simulink model "simple_router"  (R2015a)
settings: Solver=ode45  StartTime=0.0  StopTime=3000  FixedStep=1  RelTol=1e-3
undefined symbols (not defined in the file or in its folder): des, SELECT, T
libraries: simulink x16
(part 1 of 6)
settings Model: CovSFcnEnable=off  Creator=Nejib  LastModifiedBy=Nejib
settings DebuggingCC: SolverPrmCheckMsg=warning
settings SimEventsCC: propMaxDesBlkSimulEvents=100000  propMaxDesMdlSimulEvents=10000000

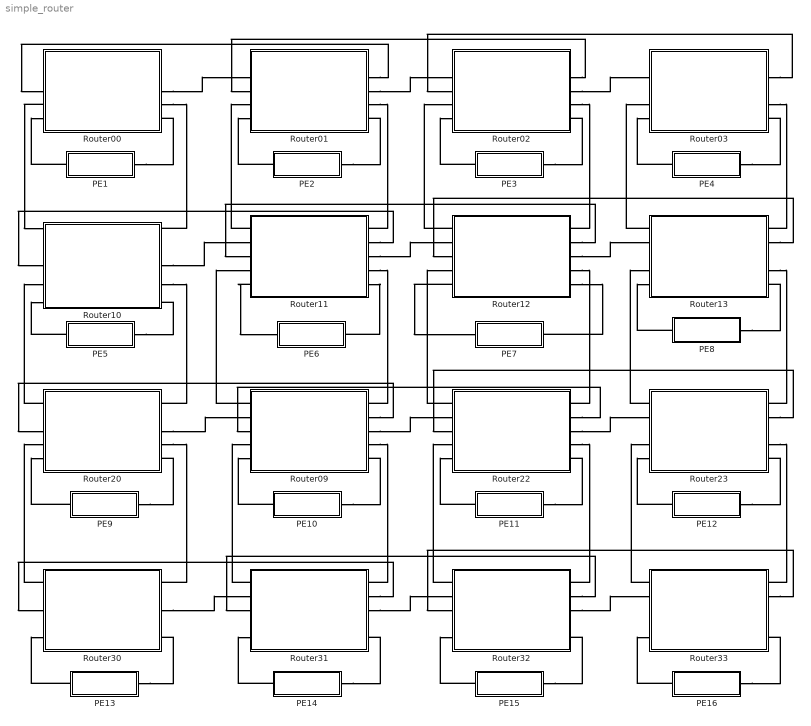
== system simple_router ==
  PE1 : Subsystem  mask{ME=1, D=5, SEED=100, tt=Periodic, MINU=10, MAXU=200, REGULAR=T, A=100, B=15, Inst='Inst1', Router='Mean1', Loss='Loss1', N='N1'}
      mask prompts: ME "Adresse"; D "Startup time"; tt "Traffic Type"; MINU "Min"; MAXU "Max"; REGULAR "T"; A "Lambda 1"; B "Lambda 2"; Inst "Instant delay"; Router "Mean delay"; Loss "Instant number of lost flits"; N "Number of departed flits"
      mask init:
      | set_param([gcb '/Inst'],'VariableName',Inst)
      | set_param([gcb '/Router'],'VariableName',Router)
      | set_param([gcb '/Loss'],'VariableName',Loss)
      | set_param([gcb '/N'],'VariableName',N)
      | V=1:16;
      | V=V(V~=ME);
      mask TypeOptions tt: Periodic | Uniform | MMPP
      mask Callback tt:
      | maskStr = get_param(gcb,'tt');
      | msk = Simulink.Mask.get(gcbh);
      | %p = msk.Parameters;
      | %
      | % P = msk.getParameter('MINU');
      | % U = msk.getParameter('MAXU');
      | % M = msk.getParameter('REGULAR');
      | 
      | P = msk.getDialogControl('Periodic');
      | U = msk.getDialogControl('Uniform');
      | M = msk.getDialogControl('MMPP');
      | 
      | % The pop-up menu is the first mask parameter.
      | %   Check the value selected in the pop-up
      | if strcmp(maskStr(1),'P'),
      | 
      |     % Set the visibility of both parameters on when
      |     %   User-defined is selected in the pop-up.
      |     %set_param(gcb,'MaskValues',{'Default','1','1'})
      |     %set_param(gcb,'MaskVisibilities','off'),
      |     SELECT = 1;
      |     P.Visible= 'on';
      |     U.Visible= 'off';
      |     M.Visible= 'off';
      | 
      | elseif strcmp(maskStr(1),'U'),
      |     P.Visible= 'off';
      |     U.Visible= 'on';
      |     M.Visible= 'off';
      | 
      |     SELECT = 2;
      | else
      |     P.Visible= 'off';
      |     U.Visible= 'off';
      |     M.Visible= 'on';
      | 
      |     SELECT = 3;
      | end
      mask DialogControl DescTextVar Prompt: Generates traffic from a given adress using one of three possible traffic patterns: Periodic, Uniform and Markov Modulated Poisson Process.
  PE10 : Subsystem  mask{ME=10, D=5, SEED=1000, tt=Periodic, MINU=10, MAXU=200, REGULAR=T, A=100, B=15, Inst='Inst10', Router='Mean10', Loss='Loss10', N='N10'}
      mask prompts: ME "Adresse"; D "Startup time"; tt "Traffic Type"; MINU "Min"; MAXU "Max"; REGULAR "T"; A "Lambda 1"; B "Lambda 2"; Inst "Instant delay"; Router "Mean delay"; Loss "Instant number of lost flits"; N "Number of departed flits"
      mask init:
      | set_param([gcb '/Inst'],'VariableName',Inst)
      | set_param([gcb '/Router'],'VariableName',Router)
      | set_param([gcb '/Loss'],'VariableName',Loss)
      | set_param([gcb '/N'],'VariableName',N)
      | V=1:16;
      | V=V(V~=ME);
      mask TypeOptions tt: Periodic | Uniform | MMPP
      mask Callback tt:
      | maskStr = get_param(gcb,'tt');
      | msk = Simulink.Mask.get(gcbh);
      | %p = msk.Parameters;
      | %
      | % P = msk.getParameter('MINU');
      | % U = msk.getParameter('MAXU');
      | % M = msk.getParameter('REGULAR');
      | 
      | P = msk.getDialogControl('Periodic');
      | U = msk.getDialogControl('Uniform');
      | M = msk.getDialogControl('MMPP');
      | 
      | % The pop-up menu is the first mask parameter.
      | %   Check the value selected in the pop-up
      | if strcmp(maskStr(1),'P'),
      | 
      |     % Set the visibility of both parameters on when
      |     %   User-defined is selected in the pop-up.
      |     %set_param(gcb,'MaskValues',{'Default','1','1'})
      |     %set_param(gcb,'MaskVisibilities','off'),
      |     SELECT = 1;
      |     P.Visible= 'on';
      |     U.Visible= 'off';
      |     M.Visible= 'off';
      | 
      | elseif strcmp(maskStr(1),'U'),
      |     P.Visible= 'off';
      |     U.Visible= 'on';
      |     M.Visible= 'off';
      | 
      |     SELECT = 2;
      | else
      |     P.Visible= 'off';
      |     U.Visible= 'off';
      |     M.Visible= 'on';
      | 
      |     SELECT = 3;
      | end
      mask DialogControl DescTextVar Prompt: Generates traffic from a given adress using one of three possible traffic patterns: Periodic, Uniform and Markov Modulated Poisson Process.
  PE11 : Subsystem  mask{ME=11, D=5, SEED=1100, tt=Periodic, MINU=10, MAXU=200, REGULAR=T, A=100, B=15, Inst='Inst11', Router='Mean11', Loss='Loss11', N='N11'}
      mask prompts: ME "Adresse"; D "Startup time"; tt "Traffic Type"; MINU "Min"; MAXU "Max"; REGULAR "T"; A "Lambda 1"; B "Lambda 2"; Inst "Instant delay"; Router "Mean delay"; Loss "Instant number of lost flits"; N "Number of departed flits"
      mask init:
      | set_param([gcb '/Inst'],'VariableName',Inst)
      | set_param([gcb '/Router'],'VariableName',Router)
      | set_param([gcb '/Loss'],'VariableName',Loss)
      | set_param([gcb '/N'],'VariableName',N)
      | V=1:16;
      | V=V(V~=ME);
      mask TypeOptions tt: Periodic | Uniform | MMPP
      mask Callback tt:
      | maskStr = get_param(gcb,'tt');
      | msk = Simulink.Mask.get(gcbh);
      | %p = msk.Parameters;
      | %
      | % P = msk.getParameter('MINU');
      | % U = msk.getParameter('MAXU');
      | % M = msk.getParameter('REGULAR');
      | 
      | P = msk.getDialogControl('Periodic');
      | U = msk.getDialogControl('Uniform');
      | M = msk.getDialogControl('MMPP');
      | 
      | % The pop-up menu is the first mask parameter.
      | %   Check the value selected in the pop-up
      | if strcmp(maskStr(1),'P'),
      | 
      |     % Set the visibility of both parameters on when
      |     %   User-defined is selected in the pop-up.
      |     %set_param(gcb,'MaskValues',{'Default','1','1'})
      |     %set_param(gcb,'MaskVisibilities','off'),
      |     SELECT = 1;
      |     P.Visible= 'on';
      |     U.Visible= 'off';
      |     M.Visible= 'off';
      | 
      | elseif strcmp(maskStr(1),'U'),
      |     P.Visible= 'off';
      |     U.Visible= 'on';
      |     M.Visible= 'off';
      | 
      |     SELECT = 2;
      | else
      |     P.Visible= 'off';
      |     U.Visible= 'off';
      |     M.Visible= 'on';
      | 
      |     SELECT = 3;
      | end
      mask DialogControl DescTextVar Prompt: Generates traffic from a given adress using one of three possible traffic patterns: Periodic, Uniform and Markov Modulated Poisson Process.
  PE12 : Subsystem  mask{ME=12, D=5, SEED=1200, tt=Periodic, MINU=10, MAXU=200, REGULAR=T, A=100, B=15, Inst='Inst12', Router='Mean12', Loss='Loss12', N='N12'}
      mask prompts: ME "Adresse"; D "Startup time"; tt "Traffic Type"; MINU "Min"; MAXU "Max"; REGULAR "T"; A "Lambda 1"; B "Lambda 2"; Inst "Instant delay"; Router "Mean delay"; Loss "Instant number of lost flits"; N "Number of departed flits"
      mask init:
      | set_param([gcb '/Inst'],'VariableName',Inst)
      | set_param([gcb '/Router'],'VariableName',Router)
      | set_param([gcb '/Loss'],'VariableName',Loss)
      | set_param([gcb '/N'],'VariableName',N)
      | V=1:16;
      | V=V(V~=ME);
      mask TypeOptions tt: Periodic | Uniform | MMPP
      mask Callback tt:
      | maskStr = get_param(gcb,'tt');
      | msk = Simulink.Mask.get(gcbh);
      | %p = msk.Parameters;
      | %
      | % P = msk.getParameter('MINU');
      | % U = msk.getParameter('MAXU');
      | % M = msk.getParameter('REGULAR');
      | 
      | P = msk.getDialogControl('Periodic');
      | U = msk.getDialogControl('Uniform');
      | M = msk.getDialogControl('MMPP');
      | 
      | % The pop-up menu is the first mask parameter.
      | %   Check the value selected in the pop-up
      | if strcmp(maskStr(1),'P'),
      | 
      |     % Set the visibility of both parameters on when
      |     %   User-defined is selected in the pop-up.
      |     %set_param(gcb,'MaskValues',{'Default','1','1'})
      |     %set_param(gcb,'MaskVisibilities','off'),
      |     SELECT = 1;
      |     P.Visible= 'on';
      |     U.Visible= 'off';
      |     M.Visible= 'off';
      | 
      | elseif strcmp(maskStr(1),'U'),
      |     P.Visible= 'off';
      |     U.Visible= 'on';
      |     M.Visible= 'off';
      | 
      |     SELECT = 2;
      | else
      |     P.Visible= 'off';
      |     U.Visible= 'off';
      |     M.Visible= 'on';
      | 
      |     SELECT = 3;
      | end
      mask DialogControl DescTextVar Prompt: Generates traffic from a given adress using one of three possible traffic patterns: Periodic, Uniform and Markov Modulated Poisson Process.
  PE13 : Subsystem  mask{ME=13, D=5, SEED=1300, tt=Periodic, MINU=10, MAXU=200, REGULAR=T, A=100, B=15, Inst='Inst13', Router='Mean13', Loss='Loss13', N='N13'}
      mask prompts: ME "Adresse"; D "Startup time"; tt "Traffic Type"; MINU "Min"; MAXU "Max"; REGULAR "T"; A "Lambda 1"; B "Lambda 2"; Inst "Instant delay"; Router "Mean delay"; Loss "Instant number of lost flits"; N "Number of departed flits"
      mask init:
      | set_param([gcb '/Inst'],'VariableName',Inst)
      | set_param([gcb '/Router'],'VariableName',Router)
      | set_param([gcb '/Loss'],'VariableName',Loss)
      | set_param([gcb '/N'],'VariableName',N)
      | V=1:16;
      | V=V(V~=ME);
      mask TypeOptions tt: Periodic | Uniform | MMPP
      mask Callback tt:
      | maskStr = get_param(gcb,'tt');
      | msk = Simulink.Mask.get(gcbh);
      | %p = msk.Parameters;
      | %
      | % P = msk.getParameter('MINU');
      | % U = msk.getParameter('MAXU');
      | % M = msk.getParameter('REGULAR');
      | 
      | P = msk.getDialogControl('Periodic');
      | U = msk.getDialogControl('Uniform');
      | M = msk.getDialogControl('MMPP');
      | 
      | % The pop-up menu is the first mask parameter.
      | %   Check the value selected in the pop-up
      | if strcmp(maskStr(1),'P'),
      | 
      |     % Set the visibility of both parameters on when
      |     %   User-defined is selected in the pop-up.
      |     %set_param(gcb,'MaskValues',{'Default','1','1'})
      |     %set_param(gcb,'MaskVisibilities','off'),
      |     SELECT = 1;
      |     P.Visible= 'on';
      |     U.Visible= 'off';
      |     M.Visible= 'off';
      | 
      | elseif strcmp(maskStr(1),'U'),
      |     P.Visible= 'off';
      |     U.Visible= 'on';
      |     M.Visible= 'off';
      | 
      |     SELECT = 2;
      | else
      |     P.Visible= 'off';
      |     U.Visible= 'off';
      |     M.Visible= 'on';
      | 
      |     SELECT = 3;
      | end
      mask DialogControl DescTextVar Prompt: Generates traffic from a given adress using one of three possible traffic patterns: Periodic, Uniform and Markov Modulated Poisson Process.
  PE14 : Subsystem  mask{ME=14, D=5, SEED=1400, tt=Periodic, MINU=10, MAXU=200, REGULAR=T, A=100, B=15, Inst='Inst14', Router='Mean14', Loss='Loss14', N='N14'}
      mask prompts: ME "Adresse"; D "Startup time"; tt "Traffic Type"; MINU "Min"; MAXU "Max"; REGULAR "T"; A "Lambda 1"; B "Lambda 2"; Inst "Instant delay"; Router "Mean delay"; Loss "Instant number of lost flits"; N "Number of departed flits"
      mask init:
      | set_param([gcb '/Inst'],'VariableName',Inst)
      | set_param([gcb '/Router'],'VariableName',Router)
      | set_param([gcb '/Loss'],'VariableName',Loss)
      | set_param([gcb '/N'],'VariableName',N)
      | V=1:16;
      | V=V(V~=ME);
      mask TypeOptions tt: Periodic | Uniform | MMPP
      mask Callback tt:
      | maskStr = get_param(gcb,'tt');
      | msk = Simulink.Mask.get(gcbh);
      | %p = msk.Parameters;
      | %
      | % P = msk.getParameter('MINU');
      | % U = msk.getParameter('MAXU');
      | % M = msk.getParameter('REGULAR');
      | 
      | P = msk.getDialogControl('Periodic');
      | U = msk.getDialogControl('Uniform');
      | M = msk.getDialogControl('MMPP');
      | 
      | % The pop-up menu is the first mask parameter.
      | %   Check the value selected in the pop-up
      | if strcmp(maskStr(1),'P'),
      | 
      |     % Set the visibility of both parameters on when
      |     %   User-defined is selected in the pop-up.
      |     %set_param(gcb,'MaskValues',{'Default','1','1'})
      |     %set_param(gcb,'MaskVisibilities','off'),
      |     SELECT = 1;
      |     P.Visible= 'on';
      |     U.Visible= 'off';
      |     M.Visible= 'off';
      | 
      | elseif strcmp(maskStr(1),'U'),
      |     P.Visible= 'off';
      |     U.Visible= 'on';
      |     M.Visible= 'off';
      | 
      |     SELECT = 2;
      | else
      |     P.Visible= 'off';
      |     U.Visible= 'off';
      |     M.Visible= 'on';
      | 
      |     SELECT = 3;
      | end
      mask DialogControl DescTextVar Prompt: Generates traffic from a given adress using one of three possible traffic patterns: Periodic, Uniform and Markov Modulated Poisson Process.
  PE15 : Subsystem  mask{ME=15, D=5, SEED=1500, tt=Periodic, MINU=10, MAXU=200, REGULAR=T, A=100, B=15, Inst='Inst15', Router='Mean15', Loss='Loss15', N='N15'}
      mask prompts: ME "Adresse"; D "Startup time"; tt "Traffic Type"; MINU "Min"; MAXU "Max"; REGULAR "T"; A "Lambda 1"; B "Lambda 2"; Inst "Instant delay"; Router "Mean delay"; Loss "Instant number of lost flits"; N "Number of departed flits"
      mask init:
      | set_param([gcb '/Inst'],'VariableName',Inst)
      | set_param([gcb '/Router'],'VariableName',Router)
      | set_param([gcb '/Loss'],'VariableName',Loss)
      | set_param([gcb '/N'],'VariableName',N)
      | V=1:16;
      | V=V(V~=ME);
      mask TypeOptions tt: Periodic | Uniform | MMPP
      mask Callback tt:
      | maskStr = get_param(gcb,'tt');
      | msk = Simulink.Mask.get(gcbh);
      | %p = msk.Parameters;
      | %
      | % P = msk.getParameter('MINU');
      | % U = msk.getParameter('MAXU');
      | % M = msk.getParameter('REGULAR');
      | 
      | P = msk.getDialogControl('Periodic');
      | U = msk.getDialogControl('Uniform');
      | M = msk.getDialogControl('MMPP');
      | 
      | % The pop-up menu is the first mask parameter.
      | %   Check the value selected in the pop-up
      | if strcmp(maskStr(1),'P'),
      | 
      |     % Set the visibility of both parameters on when
      |     %   User-defined is selected in the pop-up.
      |     %set_param(gcb,'MaskValues',{'Default','1','1'})
      |     %set_param(gcb,'MaskVisibilities','off'),
      |     SELECT = 1;
      |     P.Visible= 'on';
      |     U.Visible= 'off';
      |     M.Visible= 'off';
      | 
      | elseif strcmp(maskStr(1),'U'),
      |     P.Visible= 'off';
      |     U.Visible= 'on';
      |     M.Visible= 'off';
      | 
      |     SELECT = 2;
      | else
      |     P.Visible= 'off';
      |     U.Visible= 'off';
      |     M.Visible= 'on';
      | 
      |     SELECT = 3;
      | end
      mask DialogControl DescTextVar Prompt: Generates traffic from a given adress using one of three possible traffic patterns: Periodic, Uniform and Markov Modulated Poisson Process.
  PE16 : Subsystem  mask{ME=16, D=5, SEED=1600, tt=Periodic, MINU=10, MAXU=200, REGULAR=T, A=100, B=15, Inst='Inst16', Router='Mean16', Loss='Loss16', N='N16'}
      mask prompts: ME "Adresse"; D "Startup time"; tt "Traffic Type"; MINU "Min"; MAXU "Max"; REGULAR "T"; A "Lambda 1"; B "Lambda 2"; Inst "Instant delay"; Router "Mean delay"; Loss "Instant number of lost flits"; N "Number of departed flits"
      mask init:
      | set_param([gcb '/Inst'],'VariableName',Inst)
      | set_param([gcb '/Router'],'VariableName',Router)
      | set_param([gcb '/Loss'],'VariableName',Loss)
      | set_param([gcb '/N'],'VariableName',N)
      | V=1:16;
      | V=V(V~=ME);
      mask TypeOptions tt: Periodic | Uniform | MMPP
      mask Callback tt:
      | maskStr = get_param(gcb,'tt');
      | msk = Simulink.Mask.get(gcbh);
      | %p = msk.Parameters;
      | %
      | % P = msk.getParameter('MINU');
      | % U = msk.getParameter('MAXU');
      | % M = msk.getParameter('REGULAR');
      | 
      | P = msk.getDialogControl('Periodic');
      | U = msk.getDialogControl('Uniform');
      | M = msk.getDialogControl('MMPP');
      | 
      | % The pop-up menu is the first mask parameter.
      | %   Check the value selected in the pop-up
      | if strcmp(maskStr(1),'P'),
      | 
      |     % Set the visibility of both parameters on when
      |     %   User-defined is selected in the pop-up.
      |     %set_param(gcb,'MaskValues',{'Default','1','1'})
      |     %set_param(gcb,'MaskVisibilities','off'),
      |     SELECT = 1;
      |     P.Visible= 'on';
      |     U.Visible= 'off';
      |     M.Visible= 'off';
      | 
      | elseif strcmp(maskStr(1),'U'),
      |     P.Visible= 'off';
      |     U.Visible= 'on';
      |     M.Visible= 'off';
      | 
      |     SELECT = 2;
      | else
      |     P.Visible= 'off';
      |     U.Visible= 'off';
      |     M.Visible= 'on';
      | 
      |     SELECT = 3;
      | end
      mask DialogControl DescTextVar Prompt: Generates traffic from a given adress using one of three possible traffic patterns: Periodic, Uniform and Markov Modulated Poisson Process.
  PE2 : Subsystem  mask{ME=2, D=5, SEED=200, tt=Periodic, MINU=10, MAXU=200, REGULAR=T, A=100, B=15, Inst='Inst2', Router='Mean2', Loss='Loss2', N='N2'}
      mask prompts: ME "Adresse"; D "Startup time"; tt "Traffic Type"; MINU "Min"; MAXU "Max"; REGULAR "T"; A "Lambda 1"; B "Lambda 2"; Inst "Instant delay"; Router "Mean delay"; Loss "Instant number of lost flits"; N "Number of departed flits"
      mask init:
      | set_param([gcb '/Inst'],'VariableName',Inst)
      | set_param([gcb '/Router'],'VariableName',Router)
      | set_param([gcb '/Loss'],'VariableName',Loss)
      | set_param([gcb '/N'],'VariableName',N)
      | V=1:16;
      | V=V(V~=ME);
      mask TypeOptions tt: Periodic | Uniform | MMPP
      mask Callback tt:
      | maskStr = get_param(gcb,'tt');
      | msk = Simulink.Mask.get(gcbh);
      | %p = msk.Parameters;
      | %
      | % P = msk.getParameter('MINU');
      | % U = msk.getParameter('MAXU');
      | % M = msk.getParameter('REGULAR');
      | 
      | P = msk.getDialogControl('Periodic');
      | U = msk.getDialogControl('Uniform');
      | M = msk.getDialogControl('MMPP');
      | 
      | % The pop-up menu is the first mask parameter.
      | %   Check the value selected in the pop-up
      | if strcmp(maskStr(1),'P'),
      | 
      |     % Set the visibility of both parameters on when
      |     %   User-defined is selected in the pop-up.
      |     %set_param(gcb,'MaskValues',{'Default','1','1'})
      |     %set_param(gcb,'MaskVisibilities','off'),
      |     SELECT = 1;
      |     P.Visible= 'on';
      |     U.Visible= 'off';
      |     M.Visible= 'off';
      | 
      | elseif strcmp(maskStr(1),'U'),
      |     P.Visible= 'off';
      |     U.Visible= 'on';
      |     M.Visible= 'off';
      | 
      |     SELECT = 2;
      | else
      |     P.Visible= 'off';
      |     U.Visible= 'off';
      |     M.Visible= 'on';
      | 
      |     SELECT = 3;
      | end
      mask DialogControl DescTextVar Prompt: Generates traffic from a given adress using one of three possible traffic patterns: Periodic, Uniform and Markov Modulated Poisson Process.
  PE3 : Subsystem  mask{ME=3, D=5, SEED=300, tt=Periodic, MINU=10, MAXU=200, REGULAR=T, A=100, B=15, Inst='Inst3', Router='Mean3', Loss='Loss3', N='N3'}
      mask prompts: ME "Adresse"; D "Startup time"; tt "Traffic Type"; MINU "Min"; MAXU "Max"; REGULAR "T"; A "Lambda 1"; B "Lambda 2"; Inst "Instant delay"; Router "Mean delay"; Loss "Instant number of lost flits"; N "Number of departed flits"
      mask init:
      | set_param([gcb '/Inst'],'VariableName',Inst)
      | set_param([gcb '/Router'],'VariableName',Router)
      | set_param([gcb '/Loss'],'VariableName',Loss)
      | set_param([gcb '/N'],'VariableName',N)
      | V=1:16;
      | V=V(V~=ME);
      mask TypeOptions tt: Periodic | Uniform | MMPP
      mask Callback tt:
      | maskStr = get_param(gcb,'tt');
      | msk = Simulink.Mask.get(gcbh);
      | %p = msk.Parameters;
      | %
      | % P = msk.getParameter('MINU');
      | % U = msk.getParameter('MAXU');
      | % M = msk.getParameter('REGULAR');
      | 
      | P = msk.getDialogControl('Periodic');
      | U = msk.getDialogControl('Uniform');
      | M = msk.getDialogControl('MMPP');
      | 
      | % The pop-up menu is the first mask parameter.
      | %   Check the value selected in the pop-up
      | if strcmp(maskStr(1),'P'),
      | 
      |     % Set the visibility of both parameters on when
      |     %   User-defined is selected in the pop-up.
      |     %set_param(gcb,'MaskValues',{'Default','1','1'})
      |     %set_param(gcb,'MaskVisibilities','off'),
      |     SELECT = 1;
      |     P.Visible= 'on';
      |     U.Visible= 'off';
      |     M.Visible= 'off';
      | 
      | elseif strcmp(maskStr(1),'U'),
      |     P.Visible= 'off';
      |     U.Visible= 'on';
      |     M.Visible= 'off';
      | 
      |     SELECT = 2;
      | else
      |     P.Visible= 'off';
      |     U.Visible= 'off';
      |     M.Visible= 'on';
      | 
      |     SELECT = 3;
      | end
      mask DialogControl DescTextVar Prompt: Generates traffic from a given adress using one of three possible traffic patterns: Periodic, Uniform and Markov Modulated Poisson Process.
  PE4 : Subsystem  mask{ME=4, D=5, SEED=400, tt=Periodic, MINU=10, MAXU=200, REGULAR=T, A=100, B=15, Inst='Inst4', Router='Mean4', Loss='Loss4', N='N4'}
      mask prompts: ME "Adresse"; D "Startup time"; tt "Traffic Type"; MINU "Min"; MAXU "Max"; REGULAR "T"; A "Lambda 1"; B "Lambda 2"; Inst "Instant delay"; Router "Mean delay"; Loss "Instant number of lost flits"; N "Number of departed flits"
      mask init:
      | set_param([gcb '/Inst'],'VariableName',Inst)
      | set_param([gcb '/Router'],'VariableName',Router)
      | set_param([gcb '/Loss'],'VariableName',Loss)
      | set_param([gcb '/N'],'VariableName',N)
      | V=1:16;
      | V=V(V~=ME);
      mask TypeOptions tt: Periodic | Uniform | MMPP
      mask Callback tt:
      | maskStr = get_param(gcb,'tt');
      | msk = Simulink.Mask.get(gcbh);
      | %p = msk.Parameters;
      | %
      | % P = msk.getParameter('MINU');
      | % U = msk.getParameter('MAXU');
      | % M = msk.getParameter('REGULAR');
      | 
      | P = msk.getDialogControl('Periodic');
      | U = msk.getDialogControl('Uniform');
      | M = msk.getDialogControl('MMPP');
      | 
      | % The pop-up menu is the first mask parameter.
      | %   Check the value selected in the pop-up
      | if strcmp(maskStr(1),'P'),
      | 
      |     % Set the visibility of both parameters on when
      |     %   User-defined is selected in the pop-up.
      |     %set_param(gcb,'MaskValues',{'Default','1','1'})
      |     %set_param(gcb,'MaskVisibilities','off'),
      |     SELECT = 1;
      |     P.Visible= 'on';
      |     U.Visible= 'off';
      |     M.Visible= 'off';
      | 
      | elseif strcmp(maskStr(1),'U'),
      |     P.Visible= 'off';
      |     U.Visible= 'on';
      |     M.Visible= 'off';
      | 
      |     SELECT = 2;
      | else
      |     P.Visible= 'off';
      |     U.Visible= 'off';
      |     M.Visible= 'on';
      | 
      |     SELECT = 3;
      | end
      mask DialogControl DescTextVar Prompt: Generates traffic from a given adress using one of three possible traffic patterns: Periodic, Uniform and Markov Modulated Poisson Process.
  PE5 : Subsystem  mask{ME=5, D=5, SEED=500, tt=Periodic, MINU=10, MAXU=200, REGULAR=T, A=100, B=15, Inst='Inst5', Router='Mean5', Loss='Loss5', N='N5'}
      mask prompts: ME "Adresse"; D "Startup time"; tt "Traffic Type"; MINU "Min"; MAXU "Max"; REGULAR "T"; A "Lambda 1"; B "Lambda 2"; Inst "Instant delay"; Router "Mean delay"; Loss "Instant number of lost flits"; N "Number of departed flits"
      mask init:
      | set_param([gcb '/Inst'],'VariableName',Inst)
      | set_param([gcb '/Router'],'VariableName',Router)
      | set_param([gcb '/Loss'],'VariableName',Loss)
      | set_param([gcb '/N'],'VariableName',N)
      | V=1:16;
      | V=V(V~=ME);
      mask TypeOptions tt: Periodic | Uniform | MMPP
      mask Callback tt:
      | maskStr = get_param(gcb,'tt');
      | msk = Simulink.Mask.get(gcbh);
      | %p = msk.Parameters;
      | %
      | % P = msk.getParameter('MINU');
      | % U = msk.getParameter('MAXU');
      | % M = msk.getParameter('REGULAR');
      | 
      | P = msk.getDialogControl('Periodic');
      | U = msk.getDialogControl('Uniform');
      | M = msk.getDialogControl('MMPP');
      | 
      | % The pop-up menu is the first mask parameter.
      | %   Check the value selected in the pop-up
      | if strcmp(maskStr(1),'P'),
      | 
      |     % Set the visibility of both parameters on when
      |     %   User-defined is selected in the pop-up.
      |     %set_param(gcb,'MaskValues',{'Default','1','1'})
      |     %set_param(gcb,'MaskVisibilities','off'),
      |     SELECT = 1;
      |     P.Visible= 'on';
      |     U.Visible= 'off';
      |     M.Visible= 'off';
      | 
      | elseif strcmp(maskStr(1),'U'),
      |     P.Visible= 'off';
      |     U.Visible= 'on';
      |     M.Visible= 'off';
      | 
      |     SELECT = 2;
      | else
      |     P.Visible= 'off';
      |     U.Visible= 'off';
      |     M.Visible= 'on';
      | 
      |     SELECT = 3;
      | end
      mask DialogControl DescTextVar Prompt: Generates traffic from a given adress using one of three possible traffic patterns: Periodic, Uniform and Markov Modulated Poisson Process.
  PE6 : Subsystem  mask{ME=6, D=5, SEED=600, tt=Periodic, MINU=10, MAXU=200, REGULAR=T, A=100, B=15, Inst='Inst6', Router='Mean6', Loss='Loss6', N='N6'}
      mask prompts: ME "Adresse"; D "Startup time"; tt "Traffic Type"; MINU "Min"; MAXU "Max"; REGULAR "T"; A "Lambda 1"; B "Lambda 2"; Inst "Instant delay"; Router "Mean delay"; Loss "Instant number of lost flits"; N "Number of departed flits"
      mask init:
      | set_param([gcb '/Inst'],'VariableName',Inst)
      | set_param([gcb '/Router'],'VariableName',Router)
      | set_param([gcb '/Loss'],'VariableName',Loss)
      | set_param([gcb '/N'],'VariableName',N)
      | V=1:16;
      | V=V(V~=ME);
      mask TypeOptions tt: Periodic | Uniform | MMPP
      mask Callback tt:
      | maskStr = get_param(gcb,'tt');
      | msk = Simulink.Mask.get(gcbh);
      | %p = msk.Parameters;
      | %
      | % P = msk.getParameter('MINU');
      | % U = msk.getParameter('MAXU');
      | % M = msk.getParameter('REGULAR');
      | 
      | P = msk.getDialogControl('Periodic');
      | U = msk.getDialogControl('Uniform');
      | M = msk.getDialogControl('MMPP');
      | 
      | % The pop-up menu is the first mask parameter.
      | %   Check the value selected in the pop-up
      | if strcmp(maskStr(1),'P'),
      | 
      |     % Set the visibility of both parameters on when
      |     %   User-defined is selected in the pop-up.
      |     %set_param(gcb,'MaskValues',{'Default','1','1'})
      |     %set_param(gcb,'MaskVisibilities','off'),
      |     SELECT = 1;
      |     P.Visible= 'on';
      |     U.Visible= 'off';
      |     M.Visible= 'off';
      | 
      | elseif strcmp(maskStr(1),'U'),
      |     P.Visible= 'off';
      |     U.Visible= 'on';
      |     M.Visible= 'off';
      | 
      |     SELECT = 2;
      | else
      |     P.Visible= 'off';
      |     U.Visible= 'off';
      |     M.Visible= 'on';
      | 
      |     SELECT = 3;
      | end
      mask DialogControl DescTextVar Prompt: Generates traffic from a given adress using one of three possible traffic patterns: Periodic, Uniform and Markov Modulated Poisson Process.
  PE7 : Subsystem  mask{ME=7, D=5, SEED=700, tt=Periodic, MINU=10, MAXU=200, REGULAR=T, A=100, B=15, Inst='Inst7', Router='Mean7', Loss='Loss7', N='N7'}
      mask prompts: ME "Adresse"; D "Startup time"; tt "Traffic Type"; MINU "Min"; MAXU "Max"; REGULAR "T"; A "Lambda 1"; B "Lambda 2"; Inst "Instant delay"; Router "Mean delay"; Loss "Instant number of lost flits"; N "Number of departed flits"
      mask init:
      | set_param([gcb '/Inst'],'VariableName',Inst)
      | set_param([gcb '/Router'],'VariableName',Router)
      | set_param([gcb '/Loss'],'VariableName',Loss)
      | set_param([gcb '/N'],'VariableName',N)
      | V=1:16;
      | V=V(V~=ME);
      mask TypeOptions tt: Periodic | Uniform | MMPP
      mask Callback tt:
      | maskStr = get_param(gcb,'tt');
      | msk = Simulink.Mask.get(gcbh);
      | %p = msk.Parameters;
      | %
      | % P = msk.getParameter('MINU');
      | % U = msk.getParameter('MAXU');
      | % M = msk.getParameter('REGULAR');
      | 
      | P = msk.getDialogControl('Periodic');
      | U = msk.getDialogControl('Uniform');
      | M = msk.getDialogControl('MMPP');
      | 
      | % The pop-up menu is the first mask parameter.
      | %   Check the value selected in the pop-up
      | if strcmp(maskStr(1),'P'),
      | 
      |     % Set the visibility of both parameters on when
      |     %   User-defined is selected in the pop-up.
      |     %set_param(gcb,'MaskValues',{'Default','1','1'})
      |     %set_param(gcb,'MaskVisibilities','off'),
      |     SELECT = 1;
      |     P.Visible= 'on';
      |     U.Visible= 'off';
      |     M.Visible= 'off';
      | 
      | elseif strcmp(maskStr(1),'U'),
      |     P.Visible= 'off';
      |     U.Visible= 'on';
      |     M.Visible= 'off';
      | 
      |     SELECT = 2;
      | else
      |     P.Visible= 'off';
      |     U.Visible= 'off';
      |     M.Visible= 'on';
      | 
      |     SELECT = 3;
      | end
      mask DialogControl DescTextVar Prompt: Generates traffic from a given adress using one of three possible traffic patterns: Periodic, Uniform and Markov Modulated Poisson Process.
  PE8 : Subsystem  mask{ME=8, D=5, SEED=800, tt=Periodic, MINU=10, MAXU=200, REGULAR=T, A=100, B=15, Inst='Inst8', Router='Mean8', Loss='Loss8', N='N8'}
      mask prompts: ME "Adresse"; D "Startup time"; tt "Traffic Type"; MINU "Min"; MAXU "Max"; REGULAR "T"; A "Lambda 1"; B "Lambda 2"; Inst "Instant delay"; Router "Mean delay"; Loss "Instant number of lost flits"; N "Number of departed flits"
      mask init:
      | set_param([gcb '/Inst'],'VariableName',Inst)
      | set_param([gcb '/Router'],'VariableName',Router)
      | set_param([gcb '/Loss'],'VariableName',Loss)
      | set_param([gcb '/N'],'VariableName',N)
      | V=1:16;
      | V=V(V~=ME);
      mask TypeOptions tt: Periodic | Uniform | MMPP
      mask Callback tt:
      | maskStr = get_param(gcb,'tt');
      | msk = Simulink.Mask.get(gcbh);
      | %p = msk.Parameters;
      | %
      | % P = msk.getParameter('MINU');
      | % U = msk.getParameter('MAXU');
      | % M = msk.getParameter('REGULAR');
      | 
      | P = msk.getDialogControl('Periodic');
      | U = msk.getDialogControl('Uniform');
      | M = msk.getDialogControl('MMPP');
      | 
      | % The pop-up menu is the first mask parameter.
      | %   Check the value selected in the pop-up
      | if strcmp(maskStr(1),'P'),
      | 
      |     % Set the visibility of both parameters on when
      |     %   User-defined is selected in the pop-up.
      |     %set_param(gcb,'MaskValues',{'Default','1','1'})
      |     %set_param(gcb,'MaskVisibilities','off'),
      |     SELECT = 1;
      |     P.Visible= 'on';
      |     U.Visible= 'off';
      |     M.Visible= 'off';
      | 
      | elseif strcmp(maskStr(1),'U'),
      |     P.Visible= 'off';
      |     U.Visible= 'on';
      |     M.Visible= 'off';
      | 
      |     SELECT = 2;
      | else
      |     P.Visible= 'off';
      |     U.Visible= 'off';
      |     M.Visible= 'on';
      | 
      |     SELECT = 3;
      | end
      mask DialogControl DescTextVar Prompt: Generates traffic from a given adress using one of three possible traffic patterns: Periodic, Uniform and Markov Modulated Poisson Process.
  PE9 : Subsystem  mask{ME=9, D=5, SEED=900, tt=Periodic, MINU=10, MAXU=200, REGULAR=T, A=100, B=15, Inst='Inst9', Router='Mean9', Loss='Loss9', N='N9'}
      mask prompts: ME "Adresse"; D "Startup time"; tt "Traffic Type"; MINU "Min"; MAXU "Max"; REGULAR "T"; A "Lambda 1"; B "Lambda 2"; Inst "Instant delay"; Router "Mean delay"; Loss "Instant number of lost flits"; N "Number of departed flits"
      mask init:
      | set_param([gcb '/Inst'],'VariableName',Inst)
      | set_param([gcb '/Router'],'VariableName',Router)
      | set_param([gcb '/Loss'],'VariableName',Loss)
      | set_param([gcb '/N'],'VariableName',N)
      | V=1:16;
      | V=V(V~=ME);
      mask TypeOptions tt: Periodic | Uniform | MMPP
      mask Callback tt:
      | maskStr = get_param(gcb,'tt');
      | msk = Simulink.Mask.get(gcbh);
      | %p = msk.Parameters;
      | %
      | % P = msk.getParameter('MINU');
      | % U = msk.getParameter('MAXU');
      | % M = msk.getParameter('REGULAR');
      | 
      | P = msk.getDialogControl('Periodic');
      | U = msk.getDialogControl('Uniform');
      | M = msk.getDialogControl('MMPP');
      | 
      | % The pop-up menu is the first mask parameter.
      | %   Check the value selected in the pop-up
      | if strcmp(maskStr(1),'P'),
      | 
      |     % Set the visibility of both parameters on when
      |     %   User-defined is selected in the pop-up.
      |     %set_param(gcb,'MaskValues',{'Default','1','1'})
      |     %set_param(gcb,'MaskVisibilities','off'),
      |     SELECT = 1;
      |     P.Visible= 'on';
      |     U.Visible= 'off';
      |     M.Visible= 'off';
      | 
      | elseif strcmp(maskStr(1),'U'),
      |     P.Visible= 'off';
      |     U.Visible= 'on';
      |     M.Visible= 'off';
      | 
      |     SELECT = 2;
      | else
      |     P.Visible= 'off';
      |     U.Visible= 'off';
      |     M.Visible= 'on';
      | 
      |     SELECT = 3;
      | end
      mask DialogControl DescTextVar Prompt: Generates traffic from a given adress using one of three possible traffic patterns: Periodic, Uniform and Markov Modulated Poisson Process.
  Router00 : Subsystem  mask{ME=1, C=16, D=1, F=1, S=1e-6}
      mask prompts: ME "Router index"; C "Input FIFO size in flits"; D "Routing and arbitration delay"; F "Clock Frequency"; S "Standard Deviation"
      mask DialogControl DescTextVar Prompt: 5 Port router with the XY routing algorithm.
  Router01 : Subsystem  mask{ME=2, C=16, D=1, F=1, S=1e-6}
      mask prompts: ME "Router index"; C "Input FIFO size in flits"; D "Routing and arbitration delay"; F "Clock Frequency"; S "Standard Deviation"
      mask DialogControl DescTextVar Prompt: 5 Port router with the XY routing algorithm.
  Router02 : Subsystem  mask{ME=3, C=16, D=1e-3, F=1, S=1e-6}
      mask prompts: ME "Router index"; C "Input FIFO size in flits"; D "Routing and arbitration delay"; F "Clock Frequency"; S "Standard Deviation"
      mask DialogControl DescTextVar Prompt: 5 Port router with the XY routing algorithm.
  Router03 : Subsystem  mask{ME=4, C=16, D=1, F=1, S=1e-6}
      mask prompts: ME "Router index"; C "Input FIFO size in flits"; D "Routing and arbitration delay"; F "Clock Frequency"; S "Standard Deviation"
      mask DialogControl DescTextVar Prompt: 5 Port router with the XY routing algorithm.
  Router09 : Subsystem  mask{ME=10, C=16, D=1, F=1, S=1e-6}
      mask prompts: ME "Router index"; C "Input FIFO size in flits"; D "Routing and arbitration delay"; F "Clock Frequency"; S "Standard Deviation"
      mask DialogControl DescTextVar Prompt: 5 Port router with the XY routing algorithm.
  Router10 : Subsystem  mask{ME=5, C=16, D=1, F=1, S=1e-6}
      mask prompts: ME "Router index"; C "Input FIFO size in flits"; D "Routing and arbitration delay"; F "Clock Frequency"; S "Standard Deviation"
      mask DialogControl DescTextVar Prompt: 5 Port router with the XY routing algorithm.
  Router11 : Subsystem  mask{ME=6, C=16, D=1, F=1, S=1e-6}
      mask prompts: ME "Router index"; C "Input FIFO size in flits"; D "Routing and arbitration delay"; F "Clock Frequency"; S "Standard Deviation"
      mask DialogControl DescTextVar Prompt: 5 Port router with the XY routing algorithm.
  Router12 : Subsystem  mask{ME=7, C=16, D=1, F=1, S=1e-6}
      mask prompts: ME "Router index"; C "Input FIFO size in flits"; D "Routing and arbitration delay"; F "Clock Frequency"; S "Standard Deviation"
      mask DialogControl DescTextVar Prompt: 5 Port router with the XY routing algorithm.
  Router13 : Subsystem  mask{ME=8, C=16, D=1, F=1, S=1e-6}
      mask prompts: ME "Router index"; C "Input FIFO size in flits"; D "Routing and arbitration delay"; F "Clock Frequency"; S "Standard Deviation"
      mask DialogControl DescTextVar Prompt: 5 Port router with the XY routing algorithm.
  Router20 : Subsystem  mask{ME=9, C=16, D=1, F=1, S=1e-6}
      mask prompts: ME "Router index"; C "Input FIFO size in flits"; D "Routing and arbitration delay"; F "Clock Frequency"; S "Standard Deviation"
      mask DialogControl DescTextVar Prompt: 5 Port router with the XY routing algorithm.
  Router22 : Subsystem  mask{ME=11, C=16, D=1, F=1, S=1e-6}
      mask prompts: ME "Router index"; C "Input FIFO size in flits"; D "Routing and arbitration delay"; F "Clock Frequency"; S "Standard Deviation"
      mask DialogControl DescTextVar Prompt: 5 Port router with the XY routing algorithm.
  Router23 : Subsystem  mask{ME=12, C=16, D=1, F=1, S=1e-6}
      mask prompts: ME "Router index"; C "Input FIFO size in flits"; D "Routing and arbitration delay"; F "Clock Frequency"; S "Standard Deviation"
      mask DialogControl DescTextVar Prompt: 5 Port router with the XY routing algorithm.
  Router30 : Subsystem  mask{ME=13, C=16, D=1, F=1, S=1e-6}
      mask prompts: ME "Router index"; C "Input FIFO size in flits"; D "Routing and arbitration delay"; F "Clock Frequency"; S "Standard Deviation"
      mask DialogControl DescTextVar Prompt: 5 Port router with the XY routing algorithm.
  Router31 : Subsystem  mask{ME=14, C=16, D=1, F=1, S=1e-6}
      mask prompts: ME "Router index"; C "Input FIFO size in flits"; D "Routing and arbitration delay"; F "Clock Frequency"; S "Standard Deviation"
      mask DialogControl DescTextVar Prompt: 5 Port router with the XY routing algorithm.
  Router32 : Subsystem  mask{ME=15, C=16, D=1, F=1, S=1e-6}
      mask prompts: ME "Router index"; C "Input FIFO size in flits"; D "Routing and arbitration delay"; F "Clock Frequency"; S "Standard Deviation"
      mask DialogControl DescTextVar Prompt: 5 Port router with the XY routing algorithm.
  Router33 : Subsystem  mask{ME=16, C=16, D=1, F=1, S=1e-6}
      mask prompts: ME "Router index"; C "Input FIFO size in flits"; D "Routing and arbitration delay"; F "Clock Frequency"; S "Standard Deviation"
      mask DialogControl DescTextVar Prompt: 5 Port router with the XY routing algorithm.
  connections:
  PE1/LConn1 -- Router00/RConn5
  PE1/RConn1 -- Router00/LConn5
  PE2/RConn1 -- Router01/LConn5
  PE2/LConn1 -- Router01/RConn5
  PE3/RConn1 -- Router02/LConn5
  PE3/LConn1 -- Router02/RConn5
  PE4/RConn1 -- Router03/LConn5
  PE4/LConn1 -- Router03/RConn5
  PE5/RConn1 -- Router10/LConn5
  PE5/LConn1 -- Router10/RConn5
  Router12/LConn5 -- PE7/RConn1
  PE8/LConn1 -- Router13/RConn5
  PE8/RConn1 -- Router13/LConn5
  PE9/RConn1 -- Router20/LConn5
  PE9/LConn1 -- Router20/RConn5
  PE10/LConn1 -- Router09/RConn5
  PE10/RConn1 -- Router09/LConn5
  PE11/LConn1 -- Router22/RConn5
  PE11/RConn1 -- Router22/LConn5
  PE12/LConn1 -- Router23/RConn5
  PE12/RConn1 -- Router23/LConn5
  PE13/RConn1 -- Router30/LConn5
  PE13/LConn1 -- Router30/RConn5
  PE14/LConn1 -- Router31/RConn5
  PE14/RConn1 -- Router31/LConn5
  PE15/LConn1 -- Router32/RConn5
  PE15/RConn1 -- Router32/LConn5
  PE16/LConn1 -- Router33/RConn5
  PE16/RConn1 -- Router33/LConn5
  Router00/RConn3 -- Router01/LConn2
  Router01/RConn3 -- Router02/LConn2
  Router02/RConn3 -- Router03/LConn2
  Router10/RConn3 -- Router11/LConn2
  Router11/RConn3 -- Router12/LConn2
  Router12/RConn3 -- Router13/LConn2
  Router20/RConn3 -- Router09/LConn2
  Router09/RConn3 -- Router22/LConn2
  Router22/RConn3 -- Router23/LConn2
  Router30/RConn3 -- Router31/LConn2
  Router31/RConn3 -- Router32/LConn2
  Router32/RConn3 -- Router33/LConn2
  Router31/RConn2 -- Router30/LConn3
  Router32/RConn2 -- Router31/LConn3
  Router33/RConn2 -- Router32/LConn3
  Router09/RConn2 -- Router20/LConn3
  Router23/RConn2 -- Router22/LConn3
  Router11/RConn2 -- Router10/LConn3
  Router12/RConn2 -- Router11/LConn3
  Router13/RConn2 -- Router12/LConn3
  Router01/RConn2 -- Router00/LConn3
  Router02/RConn2 -- Router01/LConn3
  Router03/RConn2 -- Router02/LConn3
  Router01/RConn4 -- Router11/RConn1
  Router02/RConn4 -- Router12/RConn1
  Router03/RConn4 -- Router13/RConn1
  Router10/RConn4 -- Router20/RConn1
  Router11/RConn4 -- Router09/RConn1
  Router12/RConn4 -- Router22/RConn1
  Router13/RConn4 -- Router23/RConn1
  Router20/RConn4 -- Router30/RConn1
  Router22/RConn4 -- Router32/RConn1
  Router23/RConn4 -- Router33/RConn1
  Router30/LConn1 -- Router20/LConn4
  Router31/LConn1 -- Router09/LConn4
  Router22/RConn2 -- Router09/LConn3
  Router09/RConn4 -- Router31/RConn1
  Router32/LConn1 -- Router22/LConn4
  Router33/LConn1 -- Router23/LConn4
  Router23/LConn1 -- Router13/LConn4
  Router22/LConn1 -- Router12/LConn4
  Router09/LConn1 -- Router11/LConn4
  Router20/LConn1 -- Router10/LConn4
  Router11/LConn1 -- Router01/LConn4
  Router12/LConn1 -- Router02/LConn4
  Router13/LConn1 -- Router03/LConn4
  Router11/RConn5 -- PE6/LConn1
  Router11/LConn5 -- PE6/RConn1
  Router12/RConn5 -- PE7/LConn1
  Router00/RConn4 -- Router10/RConn1
  Router00/LConn4 -- Router10/LConn1

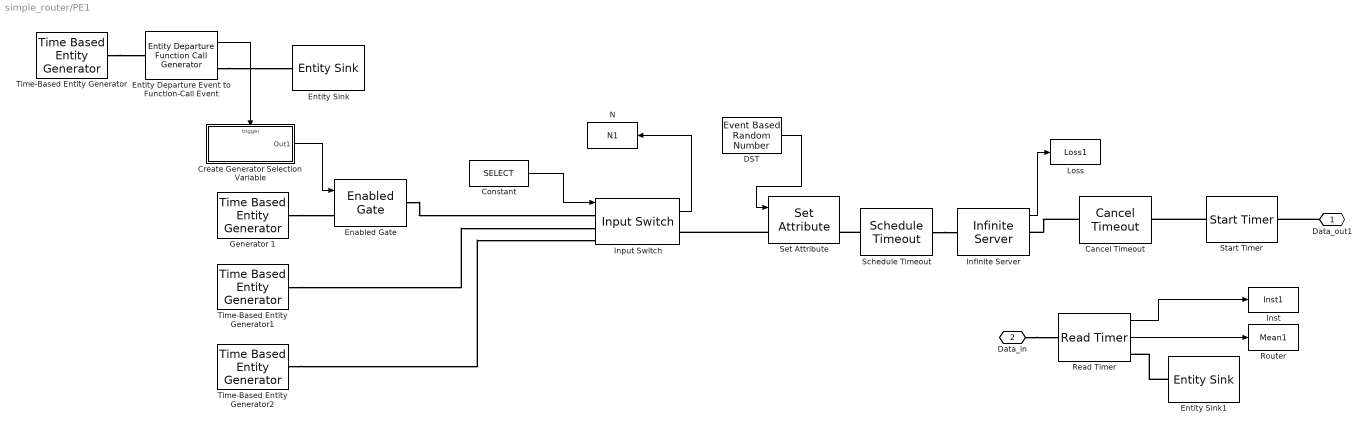
== system simple_router/PE1 ==
  Cancel Timeout : CancelTimeout
  Constant : Constant  Value=SELECT
  Create Generator Selection Variable : Subsystem  TreatAsAtomicUnit=on
      settings: PropExecContextOutsideSubsystem=on
  DST : EventBasedRandomNumber  Distribution=Arbitrary discrete  minUnid=1  maxUnid=16  numValueUnid=5  valueVecDisc=V  probVecDisc=ones(1,15)./15  Seed=SEED+5
  Enabled Gate : EnabledGate
  Entity Departure Event to Function-Call Event : EntityDepartureFunctionCallGenerator
  Entity Sink : EntitySink
  Entity Sink1 : EntitySink
  Generator 1 : TimeBasedEntityGenerator  Distribution=Exponential  Period=.1  InitialSeed=SEED+10  Maximum=.2  Mean=B  ResponseWhenUnblocked=Delayed restart  EntityType=Standard
  Infinite Server : InfiniteServer  ServiceTime=D  EnableTOPort=on  StatNumberTimedout=on
      settings: OutputPortMap=o5
  Input Switch : InputSwitch  SwitchingCriterion=From signal port p  StatNumberDeparted=on
  Inst : ToWorkspace  VariableName=Inst1  SaveFormat=Timeseries  SampleTime=-1
  Loss : ToWorkspace  VariableName=Loss1  SaveFormat=Timeseries  SampleTime=-1
  N : ToWorkspace  VariableName=N1  SaveFormat=Timeseries  SampleTime=-1
  Read Timer : ReadTimer  TimerTag=Departure  StatTimeElapsed=on  StatAverageTimeElapsed=on
      settings: OutputPortMap=o2,o3
  Router : ToWorkspace  VariableName=Mean1  SaveFormat=Timeseries  SampleTime=-1
  Schedule Timeout : ScheduleTimeout  TimeoutInterval=D
  Set Attribute : SetAttribute  AttributeName=DST|SRC  AttributeFrom=Signal port|Dialog  AttributeValue=16|1  AttributeTreatAsVector=0|0  StatNumberDeparted=on  EvaluatedAttributeValue={ [];1}
  Start Timer : StartTimer  TimerTag=Departure
  Time-Based Entity Generator : TimeBasedEntityGenerator  Distribution=Exponential  Period=15  InitialSeed=SEED  Maximum=2  Mean=A  PriorityEntityGeneration=350  EntityType=Standard
  Time-Based Entity Generator1 : TimeBasedEntityGenerator  Period=REGULAR
  Time-Based Entity Generator2 : TimeBasedEntityGenerator  Distribution=Uniform  InitialSeed=SEED  Minimum=MINU  Maximum=MAXU
  Data_out1 : PMIOPort  Port=1  Side=Right
  Data_in : PMIOPort  Port=2  Side=Left
  wires:
  Create Generator Selection Variable/1(Out1) -> Enabled Gate/1
  Entity Departure Event to Function-Call Event/1 -> Create Generator Selection Variable/Trigger
  Constant/1 -> Input Switch/1
  DST/1 -> Set Attribute/1
  Read Timer/1 -> Inst/1
  Read Timer/2 -> Router/1
  Input Switch/1 -> N/1
  Infinite Server/1 -> Loss/1
  connections:
  Entity Departure Event to Function-Call Event/RConn1 -- Entity Sink/LConn1
  Time-Based Entity Generator/RConn1 -- Entity Departure Event to Function-Call Event/LConn1
  Generator 1/RConn1 -- Enabled Gate/LConn1
  Schedule Timeout/LConn1 -- Set Attribute/RConn1
  Cancel Timeout/LConn1 -- Infinite Server/RConn1
  Set Attribute/LConn1 -- Input Switch/RConn1
  Data_out1/RConn1 -- Start Timer/RConn1
  Start Timer/LConn1 -- Cancel Timeout/RConn1
  Entity Sink1/LConn1 -- Read Timer/RConn1
  Data_in/RConn1 -- Read Timer/LConn1
  Schedule Timeout/RConn1 -- Infinite Server/LConn1
  Time-Based Entity Generator2/RConn1 -- Input Switch/LConn3
  Time-Based Entity Generator1/RConn1 -- Input Switch/LConn2
  Enabled Gate/RConn1 -- Input Switch/LConn1

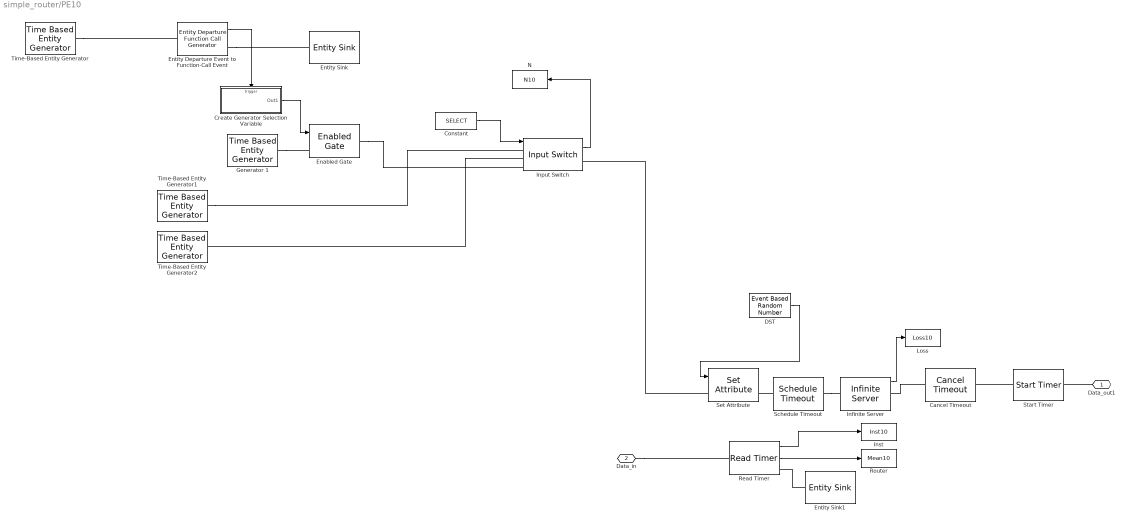
== system simple_router/PE10 ==
  Cancel Timeout : CancelTimeout
  Constant : Constant  Value=SELECT
  Create Generator Selection Variable : Subsystem  TreatAsAtomicUnit=on
      settings: PropExecContextOutsideSubsystem=on
  DST : EventBasedRandomNumber  Distribution=Arbitrary discrete  minUnid=1  maxUnid=16  numValueUnid=5  valueVecDisc=V  probVecDisc=ones(1,15)./15  Seed=SEED+5
  Enabled Gate : EnabledGate
  Entity Departure Event to Function-Call Event : EntityDepartureFunctionCallGenerator
  Entity Sink : EntitySink
  Entity Sink1 : EntitySink
  Generator 1 : TimeBasedEntityGenerator  Distribution=Exponential  Period=.1  InitialSeed=SEED+10  Maximum=.2  Mean=B  ResponseWhenUnblocked=Delayed restart  EntityType=Standard
  Infinite Server : InfiniteServer  ServiceTime=D  EnableTOPort=on  StatNumberTimedout=on
      settings: OutputPortMap=o5
  Input Switch : InputSwitch  SwitchingCriterion=From signal port p  StatNumberDeparted=on
  Inst : ToWorkspace  VariableName=Inst10  SaveFormat=Timeseries  SampleTime=-1
  Loss : ToWorkspace  VariableName=Loss10  SaveFormat=Timeseries  SampleTime=-1
  N : ToWorkspace  VariableName=N10  SaveFormat=Timeseries  SampleTime=-1
  Read Timer : ReadTimer  TimerTag=Departure  StatTimeElapsed=on  StatAverageTimeElapsed=on
      settings: OutputPortMap=o2,o3
  Router : ToWorkspace  VariableName=Mean10  SaveFormat=Timeseries  SampleTime=-1
  Schedule Timeout : ScheduleTimeout  TimeoutInterval=D
  Set Attribute : SetAttribute  AttributeName=DST|SRC  AttributeFrom=Signal port|Dialog  AttributeValue=16|1  AttributeTreatAsVector=0|0  StatNumberDeparted=on  EvaluatedAttributeValue={ [];1}
  Start Timer : StartTimer  TimerTag=Departure
  Time-Based Entity Generator : TimeBasedEntityGenerator  Distribution=Exponential  Period=15  InitialSeed=SEED  Maximum=2  Mean=A  PriorityEntityGeneration=350  EntityType=Standard
  Time-Based Entity Generator1 : TimeBasedEntityGenerator  Period=REGULAR
  Time-Based Entity Generator2 : TimeBasedEntityGenerator  Distribution=Uniform  InitialSeed=SEED  Minimum=MINU  Maximum=MAXU
  Data_out1 : PMIOPort  Port=1  Side=Right
  Data_in : PMIOPort  Port=2  Side=Left
  wires:
  Create Generator Selection Variable/1(Out1) -> Enabled Gate/1
  Entity Departure Event to Function-Call Event/1 -> Create Generator Selection Variable/Trigger
  Constant/1 -> Input Switch/1
  DST/1 -> Set Attribute/1
  Read Timer/1 -> Inst/1
  Read Timer/2 -> Router/1
  Input Switch/1 -> N/1
  Infinite Server/1 -> Loss/1
  connections:
  Entity Departure Event to Function-Call Event/RConn1 -- Entity Sink/LConn1
  Time-Based Entity Generator/RConn1 -- Entity Departure Event to Function-Call Event/LConn1
  Generator 1/RConn1 -- Enabled Gate/LConn1
  Time-Based Entity Generator1/RConn1 -- Input Switch/LConn1
  Input Switch/LConn2 -- Time-Based Entity Generator2/RConn1
  Enabled Gate/RConn1 -- Input Switch/LConn3
  Schedule Timeout/LConn1 -- Set Attribute/RConn1
  Cancel Timeout/LConn1 -- Infinite Server/RConn1
  Set Attribute/LConn1 -- Input Switch/RConn1
  Data_out1/RConn1 -- Start Timer/RConn1
  Start Timer/LConn1 -- Cancel Timeout/RConn1
  Entity Sink1/LConn1 -- Read Timer/RConn1
  Data_in/RConn1 -- Read Timer/LConn1
  Schedule Timeout/RConn1 -- Infinite Server/LConn1
